simulink model "untitled"  (R2024a)
settings: Solver=VariableStepAuto  StartTime=0.0  StopTime=100  RelTol=1e-3
values from neighbouring files (symbols this model uses):
  A = jacobian(f, [g;w])    [dynamics.m]    (also in dynamics_ext.m = jacobian(f,[w1;g1;w2;g2;w3;g3;b1;b2]); dynamics_new.m = jacobian(f,[w;g]))
  A_ext = double(subs(A,{omega11,omega12,omega13,omega21,omega22,omega23,omega31,omega32,omega33,q10,q11,q12,q13,q20,q21,q22,q23,q30,q31,q32,q33,I11,I12,I13,I21,I22,I23,I31,I32,I33,u11,u12,u13,u21,u22,u23},{w11,w12,w13,w21,w22,w23,w31,w32,w33,q10_eq,g11,g12,g13,q20_eq,g21,g22,g23,q30_eq,g31,g32,g33,i11,i12,i13,i21,i22,i23,i31,i32,i33,0,0,0,0,0,0}))    [dynamics_ext.m]
  B = jacobian(f, tau)    [dynamics.m]    (also in dynamics_ext.m = jacobian(f,[u_1;u_2]); dynamics_new.m = jacobian(f,u))
  B_ext = double(subs(B,{I11,I12,I13,I21,I22,I23,I31,I32,I33,u11,u12,u13,u21,u22,u23,omega11,omega12,omega13,omega21,omega22,omega23,omega31,omega32,omega33},{i11,i12,i13,i21,i22,i23,i31,i32,i33,0,0,0,0,0,0,w11,w12,w13,w21,w22,w23,w31,w32,w33}))    [dynamics_ext.m]
  C = eye(length(A))    [main.m]
  D = zeros(length(A),3)    [main.m]
  K = control_sys(A,B)    [main.m]
undefined symbols (not defined in the file or in its folder): C_ext, D_ext
settings Model: Creator=parid  LastModifiedBy=Floatsat
settings RTWCC: GPUComputeCapability=3.5

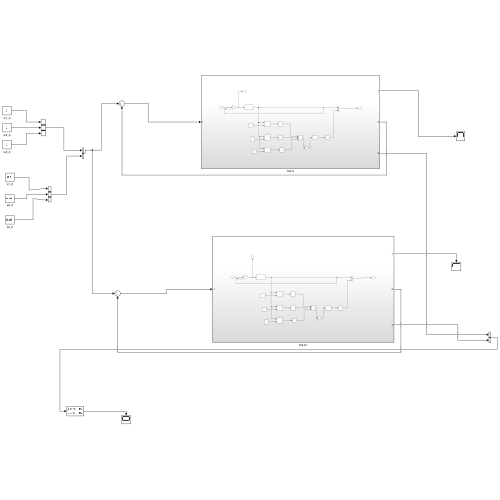
[thumbnail: Simulink's stored preview of the top-level diagram]
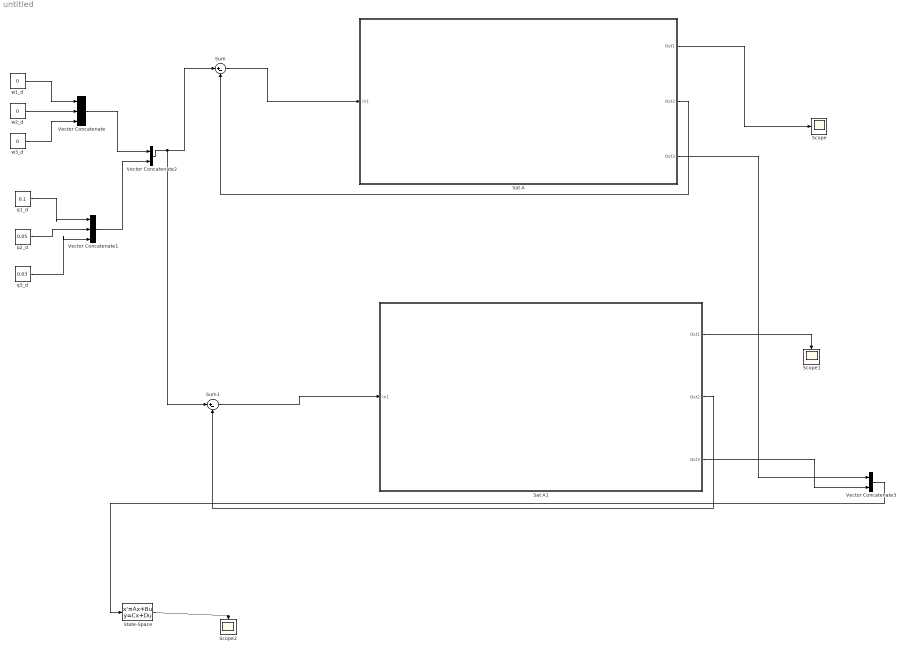
== system untitled ==
  Sat A : Subsystem
  Sat A1 : Subsystem
  Scope : Scope
  Scope1 : Scope
  Scope2 : Scope
  State-Space : StateSpace  A=A_ext  B=B_ext  C=C_ext  D=D_ext  InitialCondition=[2;2;2;0;0;0;2;2;2;0;0;0;2;2;2;0;0;0]
  Sum : Sum  Inputs=|+-
  Sum1 : Sum  Inputs=|+-
  Vector Concatenate : Concatenate  NumInputs=3
  Vector Concatenate1 : Concatenate  NumInputs=3
  Vector Concatenate2 : Concatenate
  Vector Concatenate3 : Concatenate
  q1_d : Constant  Value=0.1
  q2_d : Constant  Value=0.05
  q3_d : Constant  Value=0.03
  w1_d : Constant  Value=0
  w2_d : Constant  Value=0
  w3_d : Constant  Value=0
  wires:
  q1_d/1 -> Vector Concatenate1/1
  q2_d/1 -> Vector Concatenate1/2
  q3_d/1 -> Vector Concatenate1/3
  w1_d/1 -> Vector Concatenate/1
  w2_d/1 -> Vector Concatenate/2
  w3_d/1 -> Vector Concatenate/3
  Vector Concatenate/1 -> Vector Concatenate2/1
  Vector Concatenate1/1 -> Vector Concatenate2/2
  Vector Concatenate2/1 -> Sum1/1, Sum/1
  Sum/1 -> Sat A/1(In1)
  Sat A/1(Out1) -> Scope/1
  Sat A/2(Out2) -> Sum/2
  Sat A1/1(Out1) -> Scope1/1
  Sat A1/2(Out2) -> Sum1/2
  Sum1/1 -> Sat A1/1(In1)
  Sat A/3(Out3) -> Vector Concatenate3/1
  Sat A1/3(Out3) -> Vector Concatenate3/2
  Vector Concatenate3/1 -> State-Space/1
  State-Space/1 -> Scope2/1

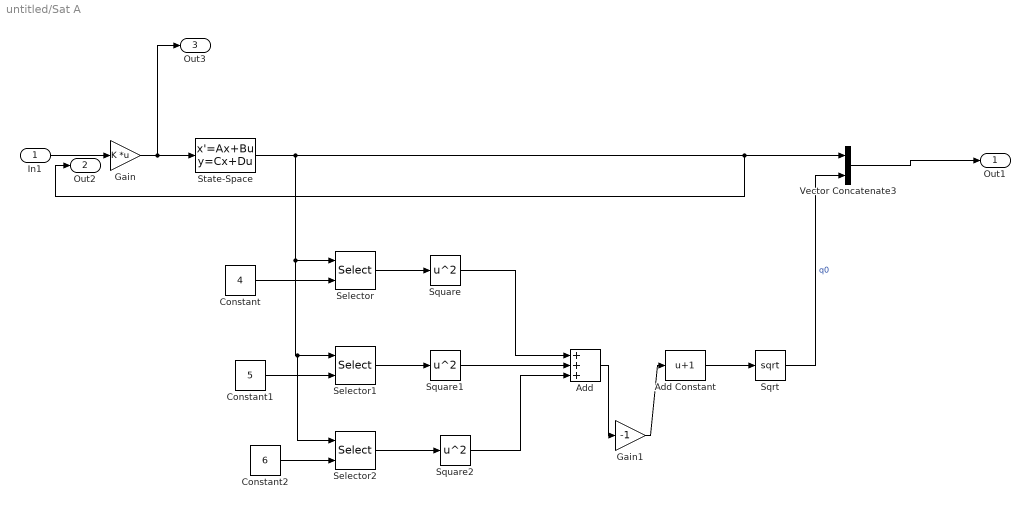
== system untitled/Sat A ==
  In1 : Inport
  Add : Sum  Inputs=+++
  Add Constant : Bias  Bias=1  SaturateOnIntegerOverflow=off
  Constant : Constant  Value=4
  Constant1 : Constant  Value=5
  Constant2 : Constant  Value=6
  Gain : Gain  Gain=K  Multiplication=Matrix(K*u)
  Gain1 : Gain  Gain=-1
  Selector : Selector  InputPortWidth=6  IndexOptions=Index vector (port)  Indices=[1 3]  OutputSizes=1
  Selector1 : Selector  InputPortWidth=6  IndexOptions=Index vector (port)  Indices=[1 3]  OutputSizes=1
  Selector2 : Selector  InputPortWidth=6  IndexOptions=Index vector (port)  Indices=[1 3]  OutputSizes=1
  Sqrt : Sqrt
  Square : Math  Operator=square
  Square1 : Math  Operator=square
  Square2 : Math  Operator=square
  State-Space : StateSpace  A=A  B=B  C=C  D=D  InitialCondition=[2;2;2;0;0;0]
  Vector Concatenate3 : Concatenate
  Out1 : Outport
  Out2 : Outport  Port=2
  Out3 : Outport  Port=3
  wires:
  State-Space/1 -> Out2/1, Vector Concatenate3/1, Selector2/1, Selector1/1, Selector/1
  Selector1/1 -> Square1/1
  Sqrt/1 -> Vector Concatenate3/2  "q0"
  Square1/1 -> Add/2
  Selector/1 -> Square/1
  Gain1/1 -> Add Constant/1
  Gain/1 -> Out3/1, State-Space/1
  Constant/1 -> Selector/2
  Selector2/1 -> Square2/1
  Add Constant/1 -> Sqrt/1
  Square/1 -> Add/1
  Constant2/1 -> Selector2/2
  Add/1 -> Gain1/1
  Constant1/1 -> Selector1/2
  Square2/1 -> Add/3
  In1/1 -> Gain/1
  Vector Concatenate3/1 -> Out1/1

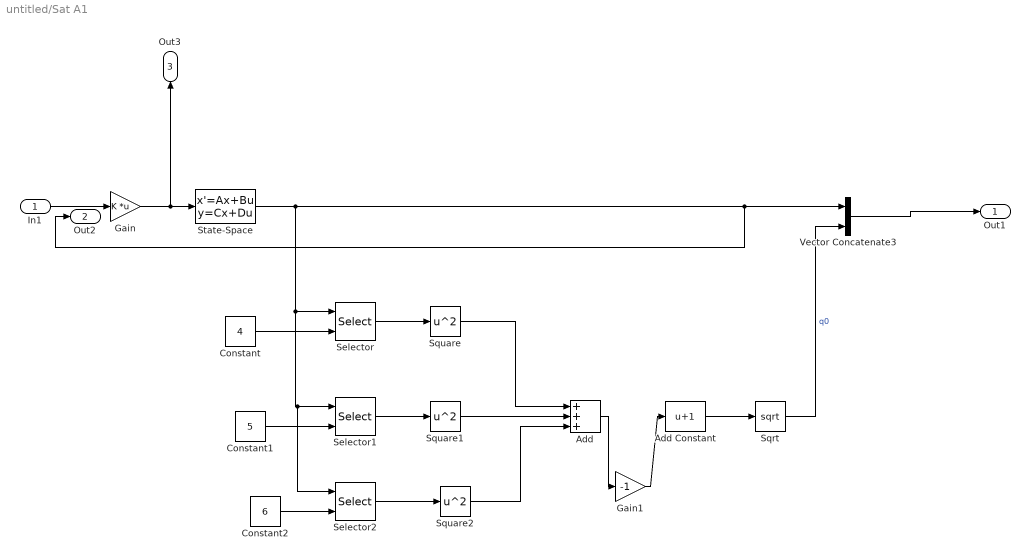
== system untitled/Sat A1 ==
  In1 : Inport
  Add : Sum  Inputs=+++
  Add Constant : Bias  Bias=1  SaturateOnIntegerOverflow=off
  Constant : Constant  Value=4
  Constant1 : Constant  Value=5
  Constant2 : Constant  Value=6
  Gain : Gain  Gain=K  Multiplication=Matrix(K*u)
  Gain1 : Gain  Gain=-1
  Selector : Selector  InputPortWidth=6  IndexOptions=Index vector (port)  Indices=[1 3]  OutputSizes=1
  Selector1 : Selector  InputPortWidth=6  IndexOptions=Index vector (port)  Indices=[1 3]  OutputSizes=1
  Selector2 : Selector  InputPortWidth=6  IndexOptions=Index vector (port)  Indices=[1 3]  OutputSizes=1
  Sqrt : Sqrt
  Square : Math  Operator=square
  Square1 : Math  Operator=square
  Square2 : Math  Operator=square
  State-Space : StateSpace  A=A  B=B  C=C  D=D  InitialCondition=[2;2;2;0;0;0]
  Vector Concatenate3 : Concatenate
  Out1 : Outport
  Out2 : Outport  Port=2
  Out3 : Outport  Port=3
  wires:
  State-Space/1 -> Out2/1, Vector Concatenate3/1, Selector2/1, Selector1/1, Selector/1
  Selector1/1 -> Square1/1
  Sqrt/1 -> Vector Concatenate3/2  "q0"
  Square1/1 -> Add/2
  Selector/1 -> Square/1
  Gain1/1 -> Add Constant/1
  Gain/1 -> Out3/1, State-Space/1
  Constant/1 -> Selector/2
  Selector2/1 -> Square2/1
  Add Constant/1 -> Sqrt/1
  Square/1 -> Add/1
  Constant2/1 -> Selector2/2
  Add/1 -> Gain1/1
  Constant1/1 -> Selector1/2
  Square2/1 -> Add/3
  In1/1 -> Gain/1
  Vector Concatenate3/1 -> Out1/1
